simulink model "memory_and_selector"  (R2020a)
settings: Solver=VariableStepAuto  StartTime=0.0  StopTime=10.0  RelTol=1e-3
libraries: hdlsllib x1
settings Model: Creator=F1  LastModifiedBy=F1

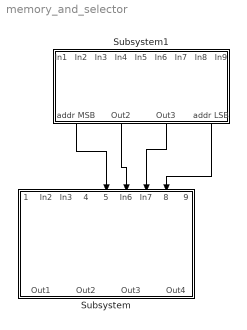
== system memory_and_selector ==
  Subsystem : Subsystem
  Subsystem1 : Subsystem
  wires:
  Subsystem1/1(addr MSB) -> Subsystem/5(addr MSB)
  Subsystem1/2(Out2) -> Subsystem/6(In6)
  Subsystem1/4(addr LSB) -> Subsystem/8(addr LSB)
  Subsystem1/3(Out3) -> Subsystem/7(In7)

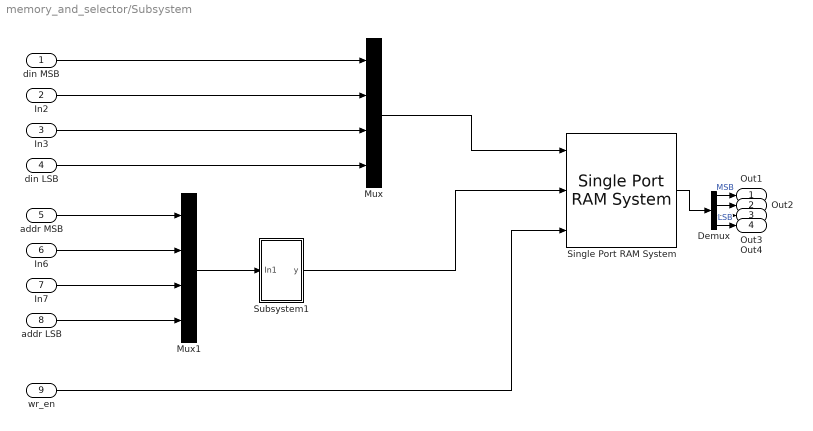
== system memory_and_selector/Subsystem ==
  din MSB : Inport
  In2 : Inport  Port=2
  In3 : Inport  Port=3
  din LSB : Inport  Port=4
  addr MSB : Inport  Port=5
  In6 : Inport  Port=6
  In7 : Inport  Port=7
  addr LSB : Inport  Port=8
  wr_en : Inport  Port=9
  Demux : Demux
  Mux : Mux
  Mux1 : Mux
  Single Port RAM System : hdlsllib/HDL RAMs/Single Port RAM System  RAMType=Single port  WriteOutputValue=New data  RAMInitialValue=0  SimulateUsing=Code generation
      settings: SourceProductBaseCode=SL
  Subsystem1 : Subsystem
  Out1 : Outport
  Out2 : Outport  Port=2
  Out3 : Outport  Port=3
  Out4 : Outport  Port=4
  wires:
  Demux/2 -> Out2/1
  Mux1/1 -> Subsystem1/1(In1)
  din LSB/1 -> Mux/4
  Demux/1 -> Out1/1  "MSB"
  Demux/3 -> Out3/1
  Subsystem1/1(y) -> Single Port RAM System/2
  Mux/1 -> Single Port RAM System/1
  Demux/4 -> Out4/1  "LSB"
  Single Port RAM System/1 -> Demux/1
  din MSB/1 -> Mux/1
  In7/1 -> Mux1/3
  addr MSB/1 -> Mux1/1
  In2/1 -> Mux/2
  In6/1 -> Mux1/2
  In3/1 -> Mux/3
  addr LSB/1 -> Mux1/4
  wr_en/1 -> Single Port RAM System/3

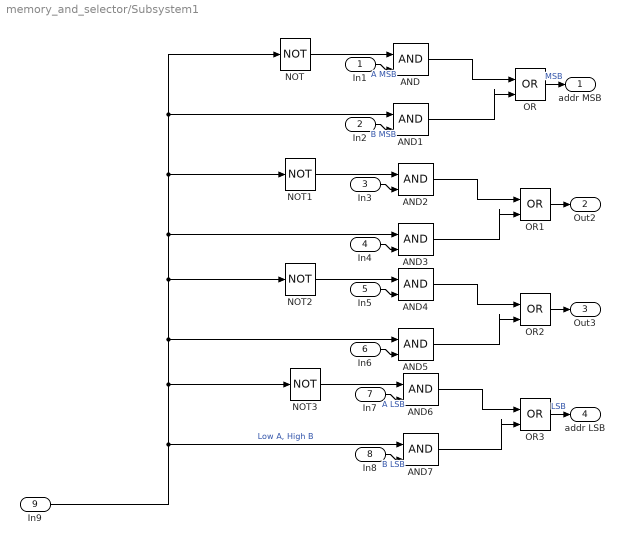
== system memory_and_selector/Subsystem1 ==
  In1 : Inport
  In2 : Inport  Port=2
  In3 : Inport  Port=3
  In4 : Inport  Port=4
  In5 : Inport  Port=5
  In6 : Inport  Port=6
  In7 : Inport  Port=7
  In8 : Inport  Port=8
  In9 : Inport  Port=9
  AND{,1..7} (8 alike) : Logic  IconShape=distinctive  AllPortsSameDT=off  OutDataTypeStr=boolean
  NOT{,1..3} (4 alike) : Logic  Operator=NOT  IconShape=distinctive  AllPortsSameDT=off  OutDataTypeStr=boolean
  OR{,1..3} (4 alike) : Logic  Operator=OR  IconShape=distinctive  AllPortsSameDT=off  OutDataTypeStr=boolean
  addr MSB : Outport
  Out2 : Outport  Port=2
  Out3 : Outport  Port=3
  addr LSB : Outport  Port=4
  wires:
  In9/1 -> AND7/1, NOT3/1, AND5/1, NOT2/1, NOT1/1, AND1/1, NOT/1, AND3/1  "Low A, High B"
  AND5/1 -> OR2/2
  NOT/1 -> AND/1
  NOT1/1 -> AND2/1
  AND/1 -> OR/1
  AND2/1 -> OR1/1
  In4/1 -> AND3/2
  NOT2/1 -> AND4/1
  AND3/1 -> OR1/2
  AND4/1 -> OR2/1
  OR1/1 -> Out2/1
  In5/1 -> AND4/2
  AND7/1 -> OR3/2
  AND1/1 -> OR/2
  OR/1 -> addr MSB/1  "MSB"
  AND6/1 -> OR3/1
  In3/1 -> AND2/2
  OR2/1 -> Out3/1
  NOT3/1 -> AND6/1
  In2/1 -> AND1/2  "B MSB"
  In6/1 -> AND5/2
  In1/1 -> AND/2  "A MSB"
  In8/1 -> AND7/2  "B LSB"
  In7/1 -> AND6/2  "A LSB"
  OR3/1 -> addr LSB/1  "LSB"

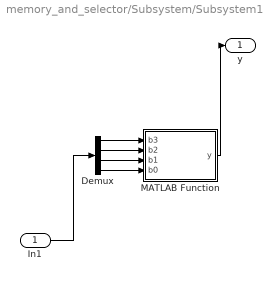
== system memory_and_selector/Subsystem/Subsystem1 ==
  In1 : Inport
  Demux : Demux
  MATLAB Function : MATLAB Function  TreatAsAtomicUnit=on
  y : Outport
  wires:
  Demux/3 -> MATLAB Function/3(b1)
  Demux/1 -> MATLAB Function/1(b3)
  Demux/2 -> MATLAB Function/2(b2)
  Demux/4 -> MATLAB Function/4(b0)
  MATLAB Function/1(y) -> y/1
  In1/1 -> Demux/1

== matlab function memory_and_selector/Subsystem/Subsystem1/MATLAB Function ==
  data: b3 input; y output; b2 input; b1 input; b0 input
function y = fcn( b3   , b2   , b1    , b0    )
y =  b3*2^3 + b2*2^2 + b1*2^1 + b0*2^0 ;
end
